simulink model "surrogate_model_2"  (R2026a)
settings: Solver=VariableStepAuto
settings Model: Creator=shuki  LastModifiedBy=shuki

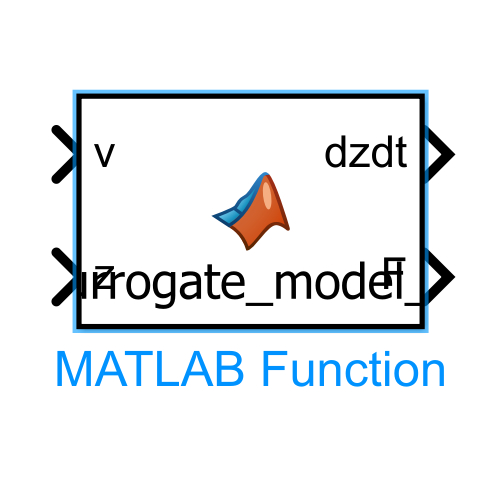
[thumbnail: Simulink's stored preview of the top-level diagram]
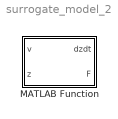
== system surrogate_model_2 ==
  MATLAB Function : MATLAB Function  TreatAsAtomicUnit=on

== matlab function surrogate_model_2/MATLAB Function ==
  data: dzdt output; F output; v input; z input
function [dzdt, F] = surrogate_model_2(v, z)

    C1 = 0.71099645;
    C2 = 5.6970253;

    dzdt = (v - (z * abs(((C1 - 10^10 * z^2)^2 * C2) - 10^5 * abs(v + z)))) + z;

    F = 10^5 * z + 316.2277 * dzdt + 0.4 * v;

end
